simulink model "Ejer13_DescomposicionPlomo"  (R2023b)
settings: Solver=FixedStepDiscrete  StartTime=0  StopTime=50  FixedStep=1  RelTol=1e-3
undefined symbols (not defined in the file): A0, B0
settings Model: Creator=alfre  LastModifiedBy=alfre

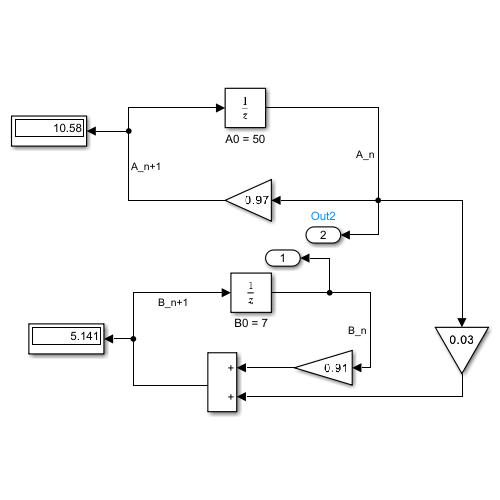
[thumbnail: Simulink's stored preview of the top-level diagram]
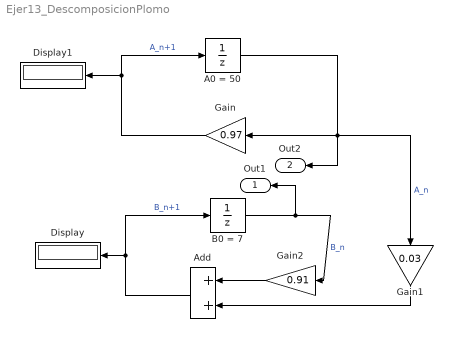
== system Ejer13_DescomposicionPlomo ==
  A0 = 50 : UnitDelay  InitialCondition=A0  SampleTime=-1  HasFrameUpgradeWarning=on
  Add : Sum
  B0 = 7 : UnitDelay  InitialCondition=B0  SampleTime=-1  HasFrameUpgradeWarning=on
  Display : Display
  Display1 : Display
  Gain : Gain  Gain=0.97
  Gain1 : Gain  Gain=0.03
  Gain2 : Gain  Gain=0.91
  Out1 : Outport
  Out2 : Outport  Port=2
  wires:
  Gain/1 -> Display1/1, A0 = 50/1  "A_n+1"
  A0 = 50/1 -> Out2/1, Gain1/1, Gain/1  "A_n"
  Add/1 -> B0 = 7/1, Display/1  "B_n+1"
  B0 = 7/1 -> Out1/1, Gain2/1  "B_n"
  Gain1/1 -> Add/2
  Gain2/1 -> Add/1
